simulink model "Computer"  (R2023a)
settings: Solver=VariableStepDiscrete  StartTime=0.0  StopTime=inf  RelTol=1e-3  EnableMultiTasking=on
values from neighbouring files (symbols this model uses):
  RomCode = Preprocessor(RomCode, c)    [ROM.m]
undefined symbols (not defined in the file or in its folder): c, in, RomCodeBreakpoints, RomData, RomDataBreakpoints, UartDataRx, UartDataRx_Active
libraries: Miscellaneous x281, simulink_extras x66, Memory_Blocks_Lib x46, simulink x42, Word_Multiplexers_Lib x31, Decoders_Lib x30, Encoders_Lib x10, Counters_Lib x9, Bit_Multiplexers_Lib x8, Arithmetic_Operations_Lib x5, Bit_Demultiplexers_Lib x4, Garbage x1
(part 4 of 6)

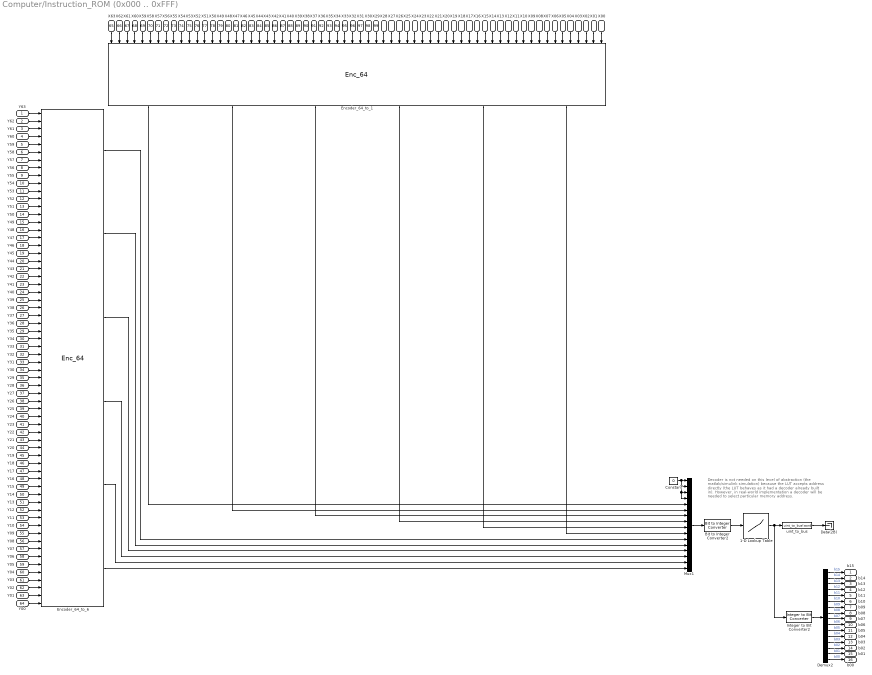
== system Computer/Instruction_ROM (0x000 .. 0xFFF) ==
  note: Decoder is not needed on this level of abstraction (the matlab/simulink simulation) because the LUT accepts address directly (the LUT behaves as it had a decoder already built in). However, in real-world implementation a decoder will be needed to select particular memory address.
  Y63 : Inport
  Y62 : Inport  Port=2
  Y61 : Inport  Port=3
  Y60 : Inport  Port=4
  Y59 : Inport  Port=5
  Y58 : Inport  Port=6
  Y57 : Inport  Port=7
  Y56 : Inport  Port=8
  Y55 : Inport  Port=9
  Y54 : Inport  Port=10
  Y53 : Inport  Port=11
  Y52 : Inport  Port=12
  Y51 : Inport  Port=13
  Y50 : Inport  Port=14
  Y49 : Inport  Port=15
  Y48 : Inport  Port=16
  Y47 : Inport  Port=17
  Y46 : Inport  Port=18
  Y45 : Inport  Port=19
  Y44 : Inport  Port=20
  Y43 : Inport  Port=21
  Y42 : Inport  Port=22
  Y41 : Inport  Port=23
  Y40 : Inport  Port=24
  Y39 : Inport  Port=25
  Y38 : Inport  Port=26
  Y37 : Inport  Port=27
  Y36 : Inport  Port=28
  Y35 : Inport  Port=29
  Y34 : Inport  Port=30
  Y33 : Inport  Port=31
  Y32 : Inport  Port=32
  Y31 : Inport  Port=33
  Y30 : Inport  Port=34
  Y29 : Inport  Port=35
  Y28 : Inport  Port=36
  Y27 : Inport  Port=37
  Y26 : Inport  Port=38
  Y25 : Inport  Port=39
  Y24 : Inport  Port=40
  Y23 : Inport  Port=41
  Y22 : Inport  Port=42
  Y21 : Inport  Port=43
  Y20 : Inport  Port=44
  Y19 : Inport  Port=45
  Y18 : Inport  Port=46
  Y17 : Inport  Port=47
  Y16 : Inport  Port=48
  Y15 : Inport  Port=49
  Y14 : Inport  Port=50
  Y13 : Inport  Port=51
  Y12 : Inport  Port=52
  Y11 : Inport  Port=53
  Y10 : Inport  Port=54
  Y09 : Inport  Port=55
  Y08 : Inport  Port=56
  Y07 : Inport  Port=57
  Y06 : Inport  Port=58
  Y05 : Inport  Port=59
  Y04 : Inport  Port=60
  Y03 : Inport  Port=61
  Y02 : Inport  Port=62
  Y01 : Inport  Port=63
  Y00 : Inport  Port=64
  X63 : Inport  Port=65
  X62 : Inport  Port=66
  X61 : Inport  Port=67
  X60 : Inport  Port=68
  X59 : Inport  Port=69
  X58 : Inport  Port=70
  X57 : Inport  Port=71
  X56 : Inport  Port=72
  X55 : Inport  Port=73
  X54 : Inport  Port=74
  X53 : Inport  Port=75
  X52 : Inport  Port=76
  X51 : Inport  Port=77
  X50 : Inport  Port=78
  X49 : Inport  Port=79
  X48 : Inport  Port=80
  X47 : Inport  Port=81
  X46 : Inport  Port=82
  X45 : Inport  Port=83
  X44 : Inport  Port=84
  X43 : Inport  Port=85
  X42 : Inport  Port=86
  X41 : Inport  Port=87
  X40 : Inport  Port=88
  X39 : Inport  Port=89
  X38 : Inport  Port=90
  X37 : Inport  Port=91
  X36 : Inport  Port=92
  X35 : Inport  Port=93
  X34 : Inport  Port=94
  X33 : Inport  Port=95
  X32 : Inport  Port=96
  X31 : Inport  Port=97
  X30 : Inport  Port=98
  X29 : Inport  Port=99
  X28 : Inport  Port=100
  X27 : Inport  Port=101
  X26 : Inport  Port=102
  X25 : Inport  Port=103
  X24 : Inport  Port=104
  X23 : Inport  Port=105
  X22 : Inport  Port=106
  X21 : Inport  Port=107
  X20 : Inport  Port=108
  X19 : Inport  Port=109
  X18 : Inport  Port=110
  X17 : Inport  Port=111
  X16 : Inport  Port=112
  X15 : Inport  Port=113
  X14 : Inport  Port=114
  X13 : Inport  Port=115
  X12 : Inport  Port=116
  X11 : Inport  Port=117
  X10 : Inport  Port=118
  X09 : Inport  Port=119
  X08 : Inport  Port=120
  X07 : Inport  Port=121
  X06 : Inport  Port=122
  X05 : Inport  Port=123
  X04 : Inport  Port=124
  X03 : Inport  Port=125
  X02 : Inport  Port=126
  X01 : Inport  Port=127
  X00 : Inport  Port=128
  1-D Lookup Table : Lookup_n-D  NumberOfTableDimensions=1  BreakpointsForDimension1=RomCodeBreakpoints  Table=RomCode  InterpMethod=Flat  InternalRulePriority=Speed  RndMeth=Simplest
  Bit to Integer Converter2 : simulink/Logic and Bit Operations/Bit to Integer Converter  nbits=16  bitOrder=MSB first  signedOutputValues=Unsigned  outDtype=uint16  outDtypeSigned=Inherit via internal rule
      settings: LibrarySourceBlock=|
      | commutil2/Bit to Integer
      | Converter
  Constant : Constant  Value=0  OutDataTypeStr=boolean
  Data(2B) : Terminator
  Demux2 : Demux  Outputs=16
  Encoder_64_to_1 : Encoders_Lib/Enc_64  SystemSampleTime=-1  VariantActivationTime=update diagram  Latency=0  AutoFrameSizeCalculation=off
      settings: LibrarySourceBlock=Garbage/Encoder_64_to_6
  Encoder_64_to_6 : Encoders_Lib/Enc_64  SystemSampleTime=-1  VariantActivationTime=update diagram  Latency=0  AutoFrameSizeCalculation=off
      settings: LibrarySourceBlock=Garbage/Encoder_64_to_6
  Integer to Bit Converter2 : simulink/Logic and Bit Operations/Integer to Bit Converter  nbits=16  signedInputValues=Unsigned  bitOrder=MSB first  outDtype=boolean
      settings: LibrarySourceBlock=|
      | commutil2/Integer to Bit
      | Converter
  Mux1 : Mux  Inputs=16
  uint_to_bus : Miscellaneous/uint_to_bus(word)
      settings: LibrarySourceBlock=Miscellaneous/uint_to_bus
  b15 : Outport
  b14 : Outport  Port=2
  b13 : Outport  Port=3
  b12 : Outport  Port=4
  b11 : Outport  Port=5
  b10 : Outport  Port=6
  b09 : Outport  Port=7
  b08 : Outport  Port=8
  b07 : Outport  Port=9
  b06 : Outport  Port=10
  b05 : Outport  Port=11
  b04 : Outport  Port=12
  b03 : Outport  Port=13
  b02 : Outport  Port=14
  b01 : Outport  Port=15
  b00 : Outport  Port=16
  wires:
  1-D Lookup Table/1 -> Integer to Bit Converter2/1, uint_to_bus/1
  Mux1/1 -> Bit to Integer Converter2/1
  uint_to_bus/1 -> Data(2B)/1
  Y04/1 -> Encoder_64_to_6/60
  Y02/1 -> Encoder_64_to_6/62
  Y57/1 -> Encoder_64_to_6/7
  Y07/1 -> Encoder_64_to_6/57
  Y22/1 -> Encoder_64_to_6/42
  Y33/1 -> Encoder_64_to_6/31
  Y54/1 -> Encoder_64_to_6/10
  Y52/1 -> Encoder_64_to_6/12
  Y39/1 -> Encoder_64_to_6/25
  Y19/1 -> Encoder_64_to_6/45
  Y60/1 -> Encoder_64_to_6/4
  Y12/1 -> Encoder_64_to_6/52
  Y44/1 -> Encoder_64_to_6/20
  Y51/1 -> Encoder_64_to_6/13
  Y58/1 -> Encoder_64_to_6/6
  Y16/1 -> Encoder_64_to_6/48
  Y11/1 -> Encoder_64_to_6/53
  Y61/1 -> Encoder_64_to_6/3
  Y32/1 -> Encoder_64_to_6/32
  Y29/1 -> Encoder_64_to_6/35
  Y15/1 -> Encoder_64_to_6/49
  Y21/1 -> Encoder_64_to_6/43
  Y03/1 -> Encoder_64_to_6/61
  Y00/1 -> Encoder_64_to_6/64
  Y23/1 -> Encoder_64_to_6/41
  Y38/1 -> Encoder_64_to_6/26
  Y05/1 -> Encoder_64_to_6/59
  Y01/1 -> Encoder_64_to_6/63
  Y06/1 -> Encoder_64_to_6/58
  Y34/1 -> Encoder_64_to_6/30
  Y08/1 -> Encoder_64_to_6/56
  Y25/1 -> Encoder_64_to_6/39
  Y36/1 -> Encoder_64_to_6/28
  Y59/1 -> Encoder_64_to_6/5
  Y40/1 -> Encoder_64_to_6/24
  Y09/1 -> Encoder_64_to_6/55
  Y42/1 -> Encoder_64_to_6/22
  Y24/1 -> Encoder_64_to_6/40
  Y62/1 -> Encoder_64_to_6/2
  Y30/1 -> Encoder_64_to_6/34
  Y53/1 -> Encoder_64_to_6/11
  Y41/1 -> Encoder_64_to_6/23
  Y35/1 -> Encoder_64_to_6/29
  Y63/1 -> Encoder_64_to_6/1
  Y48/1 -> Encoder_64_to_6/16
  Y55/1 -> Encoder_64_to_6/9
  Y13/1 -> Encoder_64_to_6/51
  Y37/1 -> Encoder_64_to_6/27
  Y45/1 -> Encoder_64_to_6/19
  Y43/1 -> Encoder_64_to_6/21
  Y50/1 -> Encoder_64_to_6/14
  Y27/1 -> Encoder_64_to_6/37
  Y49/1 -> Encoder_64_to_6/15
  Y14/1 -> Encoder_64_to_6/50
  Y18/1 -> Encoder_64_to_6/46
  Y56/1 -> Encoder_64_to_6/8
  Y26/1 -> Encoder_64_to_6/38
  Y31/1 -> Encoder_64_to_6/33
  Y20/1 -> Encoder_64_to_6/44
  Y10/1 -> Encoder_64_to_6/54
  Y17/1 -> Encoder_64_to_6/47
  Y28/1 -> Encoder_64_to_6/36
  Y47/1 -> Encoder_64_to_6/17
  Y46/1 -> Encoder_64_to_6/18
  Constant/1 -> Mux1/2, Mux1/3, Mux1/4, Mux1/1
  X63/1 -> Encoder_64_to_1/1
  X62/1 -> Encoder_64_to_1/2
  X61/1 -> Encoder_64_to_1/3
  X60/1 -> Encoder_64_to_1/4
  X59/1 -> Encoder_64_to_1/5
  X58/1 -> Encoder_64_to_1/6
  X57/1 -> Encoder_64_to_1/7
  X56/1 -> Encoder_64_to_1/8
  X55/1 -> Encoder_64_to_1/9
  X54/1 -> Encoder_64_to_1/10
  X53/1 -> Encoder_64_to_1/11
  X52/1 -> Encoder_64_to_1/12
  X51/1 -> Encoder_64_to_1/13
  X50/1 -> Encoder_64_to_1/14
  X49/1 -> Encoder_64_to_1/15
  X48/1 -> Encoder_64_to_1/16
  X47/1 -> Encoder_64_to_1/17
  X46/1 -> Encoder_64_to_1/18
  X45/1 -> Encoder_64_to_1/19
  X44/1 -> Encoder_64_to_1/20
  X43/1 -> Encoder_64_to_1/21
  X42/1 -> Encoder_64_to_1/22
  X41/1 -> Encoder_64_to_1/23
  X40/1 -> Encoder_64_to_1/24
  X39/1 -> Encoder_64_to_1/25
  X38/1 -> Encoder_64_to_1/26
  X37/1 -> Encoder_64_to_1/27
  X36/1 -> Encoder_64_to_1/28
  X35/1 -> Encoder_64_to_1/29
  X34/1 -> Encoder_64_to_1/30
  X33/1 -> Encoder_64_to_1/31
  X32/1 -> Encoder_64_to_1/32
  X31/1 -> Encoder_64_to_1/33
  X30/1 -> Encoder_64_to_1/34
  X29/1 -> Encoder_64_to_1/35
  X28/1 -> Encoder_64_to_1/36
  X27/1 -> Encoder_64_to_1/37
  X26/1 -> Encoder_64_to_1/38
  X25/1 -> Encoder_64_to_1/39
  X24/1 -> Encoder_64_to_1/40
  X23/1 -> Encoder_64_to_1/41
  X22/1 -> Encoder_64_to_1/42
  X21/1 -> Encoder_64_to_1/43
  X20/1 -> Encoder_64_to_1/44
  X19/1 -> Encoder_64_to_1/45
  X18/1 -> Encoder_64_to_1/46
  X17/1 -> Encoder_64_to_1/47
  X16/1 -> Encoder_64_to_1/48
  X15/1 -> Encoder_64_to_1/49
  X14/1 -> Encoder_64_to_1/50
  X13/1 -> Encoder_64_to_1/51
  X12/1 -> Encoder_64_to_1/52
  X11/1 -> Encoder_64_to_1/53
  X10/1 -> Encoder_64_to_1/54
  X09/1 -> Encoder_64_to_1/55
  X08/1 -> Encoder_64_to_1/56
  X07/1 -> Encoder_64_to_1/57
  X06/1 -> Encoder_64_to_1/58
  X05/1 -> Encoder_64_to_1/59
  X04/1 -> Encoder_64_to_1/60
  X03/1 -> Encoder_64_to_1/61
  X02/1 -> Encoder_64_to_1/62
  X01/1 -> Encoder_64_to_1/63
  X00/1 -> Encoder_64_to_1/64
  Bit to Integer Converter2/1 -> 1-D Lookup Table/1
  Encoder_64_to_6/6 -> Mux1/16
  Encoder_64_to_6/5 -> Mux1/15
  Encoder_64_to_6/4 -> Mux1/14
  Encoder_64_to_6/3 -> Mux1/13
  Encoder_64_to_6/2 -> Mux1/12
  Encoder_64_to_1/1 -> Mux1/5
  Encoder_64_to_1/6 -> Mux1/10
  Encoder_64_to_6/1 -> Mux1/11
  Encoder_64_to_1/5 -> Mux1/9
  Encoder_64_to_1/4 -> Mux1/8
  Encoder_64_to_1/3 -> Mux1/7
  Encoder_64_to_1/2 -> Mux1/6
  Integer to Bit Converter2/1 -> Demux2/1
  Demux2/1 -> b15/1  "b15"
  Demux2/2 -> b14/1  "b14"
  Demux2/3 -> b13/1  "b13"
  Demux2/4 -> b12/1  "b12"
  Demux2/5 -> b11/1  "b11"
  Demux2/6 -> b10/1  "b10"
  Demux2/7 -> b09/1  "b09"
  Demux2/8 -> b08/1  "b08"
  Demux2/9 -> b07/1  "b07"
  Demux2/10 -> b06/1  "b06"
  Demux2/11 -> b05/1  "b05"
  Demux2/12 -> b04/1  "b04"
  Demux2/13 -> b03/1  "b03"
  Demux2/14 -> b02/1  "b02"
  Demux2/15 -> b01/1  "b01"
  Demux2/16 -> b00/1  "b00"

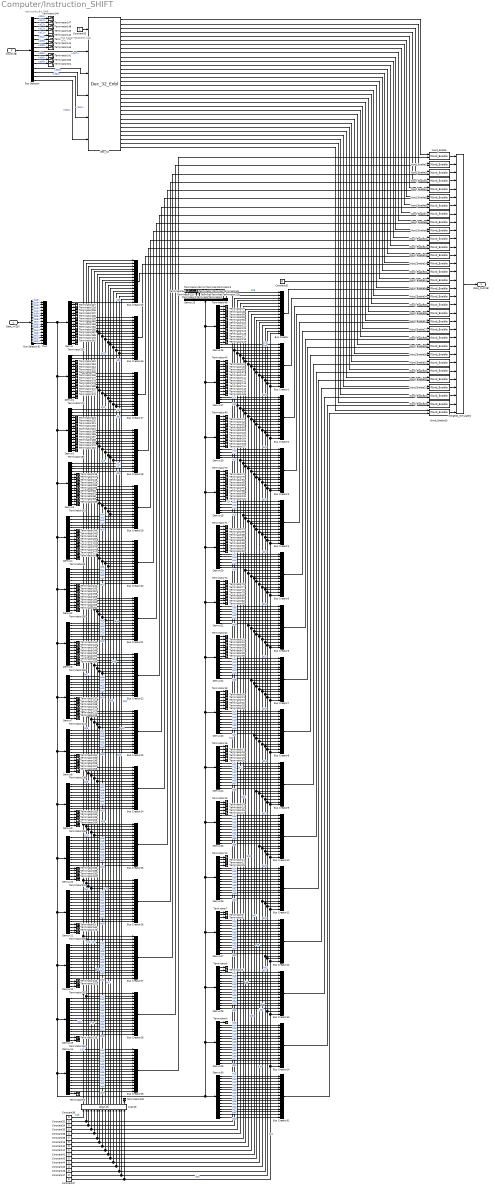
== system Computer/Instruction_SHIFT ==
  note: Instruction_Bit_Shift
  note: This signal
      | represents
      | sign (+/-).
  Data_In(2B) : Inport
  Count(2B) : Inport  Port=2
  Align16 : Miscellaneous/Align16
  Bus Creator{,1..29,31} (31 alike) : BusCreator  Inputs=16
  Bus Selector : BusSelector  OutputSignals=b15,b14,b13,b12,b11,b10,b09,b08,b07,b06,b05,b04,b03,b02,b01,b00
  Bus Selector31 : BusSelector  OutputSignals=b15,b14,b13,b12,b11,b10,b09,b08,b07,b06,b05,b04,b03,b02,b01,b00
  Constant{16,32,34..47} (16 alike) : Constant  Value=0  OutDataTypeStr=boolean
  Constant31 : Constant  Value=0  OutDataTypeStr=Bus: BUS_UINT16_T
  Constant33 : Constant  OutDataTypeStr=boolean
  Dec_32 : Decoders_Lib/Dec_32_Enbl  SystemSampleTime=-1  VariantActivationTime=update diagram  Latency=0  AutoFrameSizeCalculation=off
  Demux{,1..30} (31 alike) : Demux  Outputs=16
  Merge32_Simulated : Miscellaneous/Merge32_Simulated
      settings: LibrarySourceBlock=Memory_Blocks_Lib/Memory_Blocks_Lib/4096x1B_RAM_Simulated
  Mux : Mux  Inputs=16
  Terminator{1..129,140..145,147..153,160..214,216..221,224..272} (252 alike) : Terminator
  Word_Enable{,1..31} (32 alike) : Miscellaneous/Word_Enable  SystemSampleTime=-1  VariantActivationTime=update diagram  Latency=0  AutoFrameSizeCalculation=off
  Data_Out(2B) : Outport
  wires:
  Bus Creator14/1 -> Word_Enable23/2
  Mux/1 -> Demux1/1, Demux2/1, Demux30/1, Demux29/1, Demux24/1, Demux23/1, Demux19/1, Demux18/1, Demux17/1, Demux15/1, Demux16/1, Demux20/1, Demux21/1, Demux22/1, Demux25/1, Demux26/1, Demux27/1, Demux28/1, Demux14/1, Demux13/1, Demux12/1, Demux11/1, Demux10/1, Demux9/1, Demux8/1, Demux7/1, Demux6/1, Demux5/1, Demux4/1, Demux3/1, Demux/1
  Demux29/16 -> Bus Creator14/15  "b01"
  Demux29/15 -> Bus Creator14/14  "b02"
  Demux29/13 -> Bus Creator14/12  "b04"
  Demux29/12 -> Bus Creator14/11  "b05"
  Demux29/11 -> Bus Creator14/10  "b06"
  Demux29/10 -> Bus Creator14/9  "b07"
  Demux29/14 -> Bus Creator14/13  "b03"
  Demux29/9 -> Bus Creator14/8  "b08"
  Demux29/8 -> Bus Creator14/7  "b09"
  Demux29/7 -> Bus Creator14/6  "b10"
  Demux29/6 -> Bus Creator14/5  "b11"
  Demux29/5 -> Bus Creator14/4  "b12"
  Demux29/4 -> Bus Creator14/3  "b13"
  Demux29/3 -> Bus Creator14/2  "b14"
  Demux29/2 -> Bus Creator14/1  "b15"
  Demux29/1 -> Terminator4/1
  Demux28/16 -> Bus Creator13/14  "b02"
  Demux28/15 -> Bus Creator13/13  "b03"
  Demux28/13 -> Bus Creator13/11  "b05"
  Demux28/12 -> Bus Creator13/10  "b06"
  Demux28/11 -> Bus Creator13/9  "b07"
  Demux28/10 -> Bus Creator13/8  "b08"
  Demux28/14 -> Bus Creator13/12  "b04"
  Demux28/9 -> Bus Creator13/7  "b09"
  Demux28/8 -> Bus Creator13/6  "b10"
  Demux28/7 -> Bus Creator13/5  "b11"
  Demux28/6 -> Bus Creator13/4  "b12"
  Demux28/5 -> Bus Creator13/3  "b13"
  Demux28/4 -> Bus Creator13/2  "b14"
  Demux28/3 -> Bus Creator13/1  "b15"
  Demux28/2 -> Terminator6/1
  Demux28/1 -> Terminator5/1
  Bus Creator13/1 -> Word_Enable22/2
  Demux27/16 -> Bus Creator12/13  "b03"
  Demux27/15 -> Bus Creator12/12  "b04"
  Demux27/13 -> Bus Creator12/10  "b06"
  Demux27/12 -> Bus Creator12/9  "b07"
  Demux27/11 -> Bus Creator12/8  "b08"
  Demux27/10 -> Bus Creator12/7  "b09"
  Demux27/14 -> Bus Creator12/11  "b05"
  Demux27/9 -> Bus Creator12/6  "b10"
  Demux27/8 -> Bus Creator12/5  "b11"
  Demux27/7 -> Bus Creator12/4  "b12"
  Demux27/6 -> Bus Creator12/3  "b13"
  Demux27/5 -> Bus Creator12/2  "b14"
  Demux27/4 -> Bus Creator12/1  "b15"
  Demux27/3 -> Terminator9/1
  Demux27/2 -> Terminator8/1
  Demux27/1 -> Terminator7/1
  Bus Creator12/1 -> Word_Enable21/2
  Demux26/16 -> Bus Creator11/12  "b04"
  Demux26/15 -> Bus Creator11/11  "b05"
  Demux26/13 -> Bus Creator11/9  "b07"
  Demux26/12 -> Bus Creator11/8  "b08"
  Demux26/11 -> Bus Creator11/7  "b09"
  Demux26/10 -> Bus Creator11/6  "b10"
  Demux26/14 -> Bus Creator11/10  "b06"
  Demux26/9 -> Bus Creator11/5  "b11"
  Demux26/8 -> Bus Creator11/4  "b12"
  Demux26/7 -> Bus Creator11/3  "b13"
  Demux26/6 -> Bus Creator11/2  "b14"
  Demux26/5 -> Bus Creator11/1  "b15"
  Demux26/3 -> Terminator12/1
  Demux26/2 -> Terminator11/1
  Demux26/1 -> Terminator10/1
  Demux25/16 -> Bus Creator10/11  "b05"
  Demux25/15 -> Bus Creator10/10  "b06"
  Demux25/13 -> Bus Creator10/8  "b08"
  Demux25/12 -> Bus Creator10/7  "b09"
  Demux25/11 -> Bus Creator10/6  "b10"
  Demux25/10 -> Bus Creator10/5  "b11"
  Demux25/14 -> Bus Creator10/9  "b07"
  Demux25/9 -> Bus Creator10/4  "b12"
  Demux25/8 -> Bus Creator10/3  "b13"
  Demux25/7 -> Bus Creator10/2  "b14"
  Demux25/6 -> Bus Creator10/1  "b15"
  Demux25/5 -> Terminator27/1
  Demux25/4 -> Terminator26/1
  Demux25/3 -> Terminator15/1
  Demux25/2 -> Terminator14/1
  Demux25/1 -> Terminator13/1
  Demux24/16 -> Bus Creator9/10  "b06"
  Demux24/15 -> Bus Creator9/9  "b07"
  Demux24/13 -> Bus Creator9/7  "b09"
  Demux24/12 -> Bus Creator9/6  "b10"
  Demux24/11 -> Bus Creator9/5  "b11"
  Demux24/10 -> Bus Creator9/4  "b12"
  Demux24/14 -> Bus Creator9/8  "b08"
  Demux24/9 -> Bus Creator9/3  "b13"
  Demux24/8 -> Bus Creator9/2  "b14"
  Demux24/7 -> Bus Creator9/1  "b15"
  Demux24/6 -> Terminator30/1
  Demux24/5 -> Terminator29/1
  Demux24/4 -> Terminator28/1
  Demux24/3 -> Terminator18/1
  Demux24/2 -> Terminator17/1
  Demux24/1 -> Terminator16/1
  Demux23/16 -> Bus Creator8/9  "b07"
  Demux23/15 -> Bus Creator8/8  "b08"
  Demux23/13 -> Bus Creator8/6  "b10"
  Demux23/12 -> Bus Creator8/5  "b11"
  Demux23/11 -> Bus Creator8/4  "b12"
  Demux23/10 -> Bus Creator8/3  "b13"
  Demux23/14 -> Bus Creator8/7  "b09"
  Demux23/9 -> Bus Creator8/2  "b14"
  Demux23/8 -> Bus Creator8/1  "b15"
  Demux23/7 -> Terminator34/1
  Demux23/6 -> Terminator33/1
  Demux23/5 -> Terminator32/1
  Demux23/4 -> Terminator31/1
  Demux23/3 -> Terminator21/1
  Demux23/2 -> Terminator20/1
  Demux23/1 -> Terminator19/1
  Demux22/16 -> Bus Creator7/8  "b08"
  Demux22/15 -> Bus Creator7/7  "b09"
  Demux22/13 -> Bus Creator7/5  "b11"
  Demux22/12 -> Bus Creator7/4  "b12"
  Demux22/11 -> Bus Creator7/3  "b13"
  Demux22/10 -> Bus Creator7/2  "b14"
  Demux22/14 -> Bus Creator7/6  "b10"
  Demux22/9 -> Bus Creator7/1  "b15"
  Demux22/8 -> Terminator39/1
  Demux22/7 -> Terminator38/1
  Demux22/6 -> Terminator37/1
  Demux22/5 -> Terminator36/1
  Demux22/4 -> Terminator35/1
  Demux22/3 -> Terminator24/1
  Demux22/2 -> Terminator23/1
  Demux22/1 -> Terminator22/1
  Demux26/4 -> Terminator25/1
  Bus Creator11/1 -> Word_Enable20/2
  Bus Creator10/1 -> Word_Enable18/2
  Bus Creator9/1 -> Word_Enable31/2
  Bus Creator8/1 -> Word_Enable30/2
  Bus Creator7/1 -> Word_Enable29/2
  Demux21/16 -> Bus Creator6/7  "b09"
  Demux21/15 -> Bus Creator6/6  "b10"
  Demux21/13 -> Bus Creator6/4  "b12"
  Demux21/12 -> Bus Creator6/3  "b13"
  Demux21/11 -> Bus Creator6/2  "b14"
  Demux21/10 -> Bus Creator6/1  "b15"
  Demux21/14 -> Bus Creator6/5  "b11"
  Demux21/9 -> Terminator83/1
  Demux21/8 -> Terminator82/1
  Demux21/7 -> Terminator81/1
  Demux21/6 -> Terminator80/1
  Demux21/5 -> Terminator79/1
  Demux21/4 -> Terminator78/1
  Demux21/3 -> Terminator77/1
  Demux21/2 -> Terminator76/1
  Demux21/1 -> Terminator70/1
  Demux20/16 -> Bus Creator5/6  "b10"
  Demux20/15 -> Bus Creator5/5  "b11"
  Demux20/13 -> Bus Creator5/3  "b13"
  Demux20/12 -> Bus Creator5/2  "b14"
  Demux20/11 -> Bus Creator5/1  "b15"
  Demux20/10 -> Terminator92/1
  Demux20/14 -> Bus Creator5/4  "b12"
  Demux20/9 -> Terminator91/1
  Demux20/8 -> Terminator90/1
  Demux20/7 -> Terminator89/1
  Demux20/6 -> Terminator88/1
  Demux20/5 -> Terminator87/1
  Demux20/4 -> Terminator86/1
  Demux20/3 -> Terminator85/1
  Demux20/2 -> Terminator72/1
  Demux20/1 -> Terminator71/1
  Demux19/16 -> Bus Creator4/5  "b11"
  Demux19/15 -> Bus Creator4/4  "b12"
  Demux19/13 -> Bus Creator4/2  "b14"
  Demux19/12 -> Bus Creator4/1  "b15"
  Demux19/11 -> Terminator101/1
  Demux19/10 -> Terminator100/1
  Demux19/14 -> Bus Creator4/3  "b13"
  Demux19/9 -> Terminator99/1
  Demux19/8 -> Terminator98/1
  Demux19/7 -> Terminator97/1
  Demux19/6 -> Terminator96/1
  Demux19/5 -> Terminator95/1
  Demux19/4 -> Terminator94/1
  Demux19/3 -> Terminator75/1
  Demux19/2 -> Terminator74/1
  Demux19/1 -> Terminator73/1
  Demux18/16 -> Bus Creator3/4  "b12"
  Demux18/15 -> Bus Creator3/3  "b13"
  Demux18/13 -> Bus Creator3/1  "b15"
  Demux18/12 -> Terminator107/1
  Demux18/11 -> Terminator106/1
  Demux18/10 -> Terminator105/1
  Demux18/14 -> Bus Creator3/2  "b14"
  Demux18/9 -> Terminator104/1
  Demux18/8 -> Terminator103/1
  Demux18/7 -> Terminator102/1
  Demux18/6 -> Terminator93/1
  Demux18/5 -> Terminator84/1
  Demux18/3 -> Terminator42/1
  Demux18/2 -> Terminator41/1
  Demux18/1 -> Terminator40/1
  Demux17/16 -> Bus Creator2/3  "b13"
  Demux17/15 -> Bus Creator2/2  "b14"
  Demux17/13 -> Terminator109/1
  Demux17/12 -> Terminator108/1
  Demux17/11 -> Terminator115/1
  Demux17/10 -> Terminator114/1
  Demux17/14 -> Bus Creator2/1  "b15"
  Demux17/9 -> Terminator113/1
  Demux17/8 -> Terminator112/1
  Demux17/7 -> Terminator111/1
  Demux17/6 -> Terminator110/1
  Demux17/5 -> Terminator57/1
  Demux17/4 -> Terminator56/1
  Demux17/3 -> Terminator45/1
  Demux17/2 -> Terminator44/1
  Demux17/1 -> Terminator43/1
  Demux16/16 -> Bus Creator1/2  "b14"
  Demux16/15 -> Bus Creator1/1  "b15"
  Demux16/13 -> Terminator118/1
  Demux16/12 -> Terminator117/1
  Demux16/11 -> Terminator116/1
  Demux16/10 -> Terminator124/1
  Demux16/14 -> Terminator119/1
  Demux16/9 -> Terminator123/1
  Demux16/8 -> Terminator122/1
  Demux16/7 -> Terminator121/1
  Demux16/6 -> Terminator60/1
  Demux16/5 -> Terminator59/1
  Demux16/4 -> Terminator58/1
  Demux16/3 -> Terminator48/1
  Demux16/2 -> Terminator47/1
  Demux16/1 -> Terminator46/1
  Demux14/16 -> Terminator52/1
  Demux18/4 -> Terminator55/1
  Bus Creator6/1 -> Word_Enable28/2
  Bus Creator5/1 -> Word_Enable27/2
  Bus Creator4/1 -> Word_Enable17/2
  Bus Creator3/1 -> Word_Enable26/2
  Bus Creator2/1 -> Word_Enable25/2
  Bus Creator1/1 -> Word_Enable24/2
  Bus Creator/1 -> Word_Enable16/2
  Bus Creator29/1 -> Word_Enable/2
  Bus Creator28/1 -> Word_Enable2/2
  Bus Creator27/1 -> Word_Enable3/2
  Bus Creator26/1 -> Word_Enable4/2
  Bus Creator25/1 -> Word_Enable1/2
  Bus Creator24/1 -> Word_Enable5/2
  Bus Creator23/1 -> Word_Enable6/2
  Bus Creator22/1 -> Word_Enable7/2
  Bus Creator21/1 -> Word_Enable8/2
  Bus Creator20/1 -> Word_Enable9/2
  Bus Creator19/1 -> Word_Enable10/2
  Bus Creator18/1 -> Word_Enable12/2
  Bus Creator17/1 -> Word_Enable13/2
  Bus Creator16/1 -> Word_Enable14/2
  Bus Creator15/1 -> Word_Enable15/2
  Constant31/1 -> Word_Enable11/2
  Data_In(2B)/1 -> Bus Selector31/1
  Bus Selector31/1 -> Mux/1  "<b15>"
  Bus Selector31/2 -> Mux/2  "<b14>"
  Bus Selector31/4 -> Mux/4  "<b12>"
  Bus Selector31/3 -> Mux/3  "<b13>"
  Bus Selector31/5 -> Mux/5  "<b11>"
  Bus Selector31/6 -> Mux/6  "<b10>"
  Bus Selector31/7 -> Mux/7  "<b09>"
  Bus Selector31/8 -> Mux/8  "<b08>"
  Bus Selector31/9 -> Mux/9  "<b07>"
  Bus Selector31/10 -> Mux/10  "<b06>"
  Bus Selector31/11 -> Mux/11  "<b05>"
  Bus Selector31/12 -> Mux/12  "<b04>"
  Bus Selector31/13 -> Mux/13  "<b03>"
  Bus Selector31/14 -> Mux/14  "<b02>"
  Bus Selector31/15 -> Mux/15  "<b01>"
  Bus Selector31/16 -> Mux/16  "<b00>"
  Demux30/1 -> Bus Creator31/1  "b15"
  Demux30/2 -> Bus Creator31/2  "b14"
  Demux30/4 -> Bus Creator31/4  "b12"
  Demux30/3 -> Bus Creator31/3  "b13"
  Demux30/5 -> Bus Creator31/5  "b11"
  Demux30/6 -> Bus Creator31/6  "b10"
  Demux30/7 -> Bus Creator31/7  "b09"
  Demux30/8 -> Bus Creator31/8  "b08"
  Demux30/9 -> Bus Creator31/9  "b07"
  Demux30/10 -> Bus Creator31/10  "b06"
  Demux30/11 -> Bus Creator31/11  "b05"
  Demux30/12 -> Bus Creator31/12  "b04"
  Demux30/13 -> Bus Creator31/13  "b03"
  Demux30/14 -> Bus Creator31/14  "b02"
  Demux30/15 -> Bus Creator31/15  "b01"
  Demux30/16 -> Bus Creator31/16  "b00"
  Bus Creator31/1 -> Word_Enable19/2
  Dec_32/32 -> Word_Enable19/1
  Dec_32/31 -> Word_Enable23/1
  Dec_32/30 -> Word_Enable22/1
  Dec_32/29 -> Word_Enable21/1
  Dec_32/28 -> Word_Enable20/1
  Dec_32/27 -> Word_Enable18/1
  Dec_32/26 -> Word_Enable31/1
  Dec_32/25 -> Word_Enable30/1
  Dec_32/24 -> Word_Enable29/1
  Dec_32/23 -> Word_Enable28/1
  Dec_32/22 -> Word_Enable27/1
  Dec_32/21 -> Word_Enable17/1
  Dec_32/20 -> Word_Enable26/1
  Dec_32/19 -> Word_Enable25/1
  Dec_32/18 -> Word_Enable24/1
  Dec_32/17 -> Word_Enable16/1
  Dec_32/1 -> Word_Enable/1
  Dec_32/2 -> Word_Enable2/1
  Dec_32/3 -> Word_Enable3/1
  Dec_32/4 -> Word_Enable4/1
  Dec_32/5 -> Word_Enable1/1
  Dec_32/6 -> Word_Enable5/1
  Dec_32/7 -> Word_Enable6/1
  Dec_32/8 -> Word_Enable7/1
  Dec_32/9 -> Word_Enable8/1
  Dec_32/10 -> Word_Enable9/1
  Dec_32/11 -> Word_Enable10/1
  Dec_32/12 -> Word_Enable12/1
  Dec_32/13 -> Word_Enable13/1
  Dec_32/14 -> Word_Enable14/1
  Dec_32/15 -> Word_Enable15/1
  Dec_32/16 -> Word_Enable11/1
  Constant47/1 -> Align16/15, Bus Creator12/15, Bus Creator11/15, Bus Creator10/15, Bus Creator9/15, Bus Creator8/15, Bus Creator7/15, Bus Creator6/15, Bus Creator5/15, Bus Creator4/15, Bus Creator3/15, Bus Creator2/15, Bus Creator1/15, Bus Creator/15, Bus Creator13/15  "b01"
  Constant42/1 -> Align16/10, Bus Creator8/10, Bus Creator7/10, Bus Creator6/10, Bus Creator5/10, Bus Creator4/10, Bus Creator3/10, Bus Creator2/10, Bus Creator1/10, Bus Creator/10  "b06"
  Constant32/1 -> Align16/2, Bus Creator/2  "b14"
  Constant40/1 -> Align16/8, Bus Creator6/8, Bus Creator5/8, Bus Creator4/8, Bus Creator3/8, Bus Creator2/8, Bus Creator1/8, Bus Creator/8  "b08"
  Constant39/1 -> Align16/6, Bus Creator4/6, Bus Creator3/6, Bus Creator2/6, Bus Creator1/6, Bus Creator/6  "b10"
  Constant41/1 -> Align16/9, Bus Creator7/9, Bus Creator6/9, Bus Creator5/9, Bus Creator4/9, Bus Creator3/9, Bus Creator2/9, Bus Creator1/9, Bus Creator/9  "b07"
  Constant34/1 -> Align16/3, Bus Creator1/3, Bus Creator/3  "b13"
  Constant37/1 -> Align16/16, Bus Creator14/16, Bus Creator12/16, Bus Creator11/16, Bus Creator10/16, Bus Creator9/16, Bus Creator8/16, Bus Creator7/16, Bus Creator6/16, Bus Creator5/16, Bus Creator4/16, Bus Creator3/16, Bus Creator2/16, Bus Creator1/16, Bus Creator/16, Bus Creator13/16  "b00"
  Constant38/1 -> Align16/5, Bus Creator3/5, Bus Creator2/5, Bus Creator1/5, Bus Creator/5  "b11"
  Constant35/1 -> Align16/4, Bus Creator2/4, Bus Creator1/4, Bus Creator/4  "b12"
  Constant16/1 -> Align16/7, Bus Creator5/7, Bus Creator4/7, Bus Creator3/7, Bus Creator2/7, Bus Creator1/7, Bus Creator/7  "b09"
  Constant43/1 -> Align16/11, Bus Creator9/11, Bus Creator8/11, Bus Creator7/11, Bus Creator6/11, Bus Creator5/11, Bus Creator4/11, Bus Creator3/11, Bus Creator2/11, Bus Creator1/11, Bus Creator/11  "b05"
  Constant44/1 -> Align16/12, Bus Creator10/12, Bus Creator9/12, Bus Creator8/12, Bus Creator7/12, Bus Creator6/12, Bus Creator5/12, Bus Creator4/12, Bus Creator3/12, Bus Creator2/12, Bus Creator/12, Bus Creator1/12  "b04"
  Constant46/1 -> Align16/14, Bus Creator12/14, Bus Creator11/14, Bus Creator10/14, Bus Creator9/14, Bus Creator8/14, Bus Creator7/14, Bus Creator6/14, Bus Creator5/14, Bus Creator4/14, Bus Creator3/14, Bus Creator2/14, Bus Creator1/14, Bus Creator/14  "b02"
  Constant45/1 -> Align16/13, Bus Creator11/13, Bus Creator10/13, Bus Creator9/13, Bus Creator8/13, Bus Creator7/13, Bus Creator6/13, Bus Creator5/13, Bus Creator4/13, Bus Creator3/13, Bus Creator2/13, Bus Creator1/13, Bus Creator/13  "b03"
  Demux15/7 -> Terminator50/1
  Demux15/1 -> Terminator63/1
  Demux15/6 -> Terminator127/1
  Demux15/5 -> Terminator126/1
  Demux15/4 -> Terminator125/1
  Demux15/10 -> Terminator62/1
  Demux15/11 -> Terminator1/1
  Demux15/12 -> Terminator2/1
  Demux15/8 -> Terminator51/1
  Demux15/2 -> Terminator64/1
  Demux15/9 -> Terminator61/1
  Demux15/14 -> Terminator49/1
  Demux15/3 -> Terminator120/1
  Demux15/13 -> Terminator3/1
  Demux15/15 -> Terminator128/1
  Demux15/16 -> Bus Creator/1  "b15"
  Demux14/7 -> Bus Creator29/8  "b08"
  Demux10/9 -> Bus Creator25/14  "b02"
  Align16/15 -> Bus Creator15/15  "b01"
  Align16/4 -> Bus Creator25/4, Bus Creator24/4, Bus Creator23/4, Bus Creator22/4, Bus Creator21/4, Bus Creator20/4, Bus Creator19/4, Bus Creator18/4, Bus Creator17/4, Bus Creator16/4, Bus Creator15/4, Bus Creator26/4  "b12"
  Demux10/2 -> Bus Creator25/7  "b09"
  Demux8/10 -> Terminator194/1
  Demux6/1 -> Bus Creator21/10  "b06"
  Demux5/15 -> Terminator264/1
  Demux6/6 -> Bus Creator21/15  "b01"
  Demux6/5 -> Bus Creator21/14  "b02"
  Demux13/12 -> Bus Creator28/14  "b02"
  Demux11/7 -> Bus Creator26/11  "b05"
  Demux7/2 -> Bus Creator22/10  "b06"
  Demux7/14 -> Terminator212/1
  Demux8/4 -> Bus Creator23/11  "b05"
  Demux8/2 -> Bus Creator23/9  "b07"
  Demux12/8 -> Bus Creator27/11  "b05"
  Demux7/12 -> Terminator210/1
  Demux7/15 -> Terminator213/1
  Demux6/14 -> Terminator253/1
  Demux7/16 -> Terminator214/1
  Demux8/12 -> Terminator196/1
  Demux13/1 -> Bus Creator28/3  "b13"
  Align16/14 -> Bus Creator16/14, Bus Creator15/14  "b02"
  Demux9/8 -> Bus Creator24/14  "b02"
  Demux9/14 -> Terminator203/1
  Demux9/5 -> Bus Creator24/11  "b05"
  Demux9/11 -> Terminator191/1
  Demux6/11 -> Terminator249/1
  Demux9/13 -> Terminator193/1
  Demux9/15 -> Terminator204/1
  Demux10/6 -> Bus Creator25/11  "b05"
  Demux10/1 -> Bus Creator25/6  "b10"
  Demux10/10 -> Bus Creator25/15  "b01"
  Demux10/8 -> Bus Creator25/13  "b03"
  Demux12/2 -> Bus Creator27/5  "b11"
  Demux11/11 -> Bus Creator26/15  "b01"
  Demux11/6 -> Bus Creator26/10  "b06"
  Demux12/14 -> Terminator240/1
  Demux13/13 -> Bus Creator28/15  "b01"
  Demux12/5 -> Bus Creator27/8  "b08"
  Demux10/11 -> Bus Creator25/16  "b00"
  Demux10/13 -> Terminator189/1
  Demux3/1 -> Bus Creator18/13  "b03"
  Demux11/5 -> Bus Creator26/9  "b07"
  Demux11/10 -> Bus Creator26/14  "b02"
  Demux12/6 -> Bus Creator27/9  "b07"
  Demux2/5 -> Terminator220/1
  Demux2/3 -> Bus Creator17/16  "b00"
  Demux1/10 -> Terminator178/1
  Demux1/15 -> Terminator173/1
  Demux1/14 -> Terminator172/1
  Demux6/7 -> Bus Creator21/16  "b00"
  Demux12/12 -> Bus Creator27/15  "b01"
  Demux6/15 -> Terminator254/1
  Demux1/16 -> Terminator174/1
  Demux2/16 -> Terminator163/1
  Demux7/9 -> Terminator197/1
  Demux2/12 -> Terminator168/1
  Demux2/15 -> Terminator162/1
  Demux10/5 -> Bus Creator25/10  "b06"
  Demux2/9 -> Terminator165/1
  Demux2/11 -> Terminator167/1
  Demux3/2 -> Bus Creator18/14  "b02"
  Demux6/4 -> Bus Creator21/13  "b03"
  Demux6/2 -> Bus Creator21/11  "b05"
  Demux9/7 -> Bus Creator24/13  "b03"
  Demux3/7 -> Terminator218/1
  Demux3/8 -> Terminator229/1
  Demux6/16 -> Terminator255/1
  Demux3/14 -> Terminator69/1
  Demux3/16 -> Terminator161/1
  Demux3/11 -> Terminator66/1
  Demux4/7 -> Terminator245/1
  Demux3/12 -> Terminator67/1
  Demux7/3 -> Bus Creator22/11  "b05"
  Demux3/10 -> Terminator266/1
  Demux3/13 -> Terminator68/1
  Demux4/4 -> Bus Creator19/15  "b01"
  Demux9/2 -> Bus Creator24/8  "b08"
  Demux4/2 -> Bus Creator19/13  "b03"
  Demux14/13 -> Bus Creator29/14  "b02"
  Demux4/3 -> Bus Creator19/14  "b02"
  Demux4/8 -> Terminator246/1
  Demux4/5 -> Bus Creator19/16  "b00"
  Demux5/1 -> Bus Creator20/11  "b05"
  Demux7/5 -> Bus Creator22/13  "b03"
  Demux4/6 -> Terminator244/1
  Align16/3 -> Bus Creator26/3, Bus Creator25/3, Bus Creator24/3, Bus Creator23/3, Bus Creator22/3, Bus Creator21/3, Bus Creator20/3, Bus Creator19/3, Bus Creator18/3, Bus Creator17/3, Bus Creator16/3, Bus Creator15/3, Bus Creator27/3  "b13"
  Demux11/9 -> Bus Creator26/13  "b03"
  Demux5/5 -> Bus Creator20/15  "b01"
  Demux7/1 -> Bus Creator22/9  "b07"
  Demux6/9 -> Terminator247/1
  Demux5/8 -> Terminator243/1
  Demux9/1 -> Bus Creator24/7  "b09"
  Demux5/9 -> Terminator257/1
  Demux7/10 -> Terminator198/1
  Demux10/16 -> Terminator202/1
  Demux5/13 -> Terminator261/1
  Demux8/5 -> Bus Creator23/12  "b04"
  Demux3/9 -> Terminator256/1
  Demux11/8 -> Bus Creator26/12  "b04"
  Align16/5 -> Bus Creator25/5, Bus Creator24/5, Bus Creator23/5, Bus Creator22/5, Bus Creator21/5, Bus Creator20/5, Bus Creator19/5, Bus Creator18/5, Bus Creator17/5, Bus Creator16/5, Bus Creator15/5  "b11"
  Demux1/2 -> Bus Creator16/16  "b00"
  Demux1/4 -> Terminator153/1
  Demux14/6 -> Bus Creator29/7  "b09"
  Demux2/2 -> Bus Creator17/15  "b01"
  Demux8/13 -> Terminator206/1
  Demux4/9 -> Terminator267/1
  Demux12/3 -> Bus Creator27/6  "b10"
  Demux/12 -> Terminator187/1
  Demux1/13 -> Terminator171/1
  Demux2/4 -> Terminator219/1
  Demux12/11 -> Bus Creator27/14  "b02"
  Demux4/11 -> Terminator269/1
  Demux1/12 -> Terminator180/1
  Demux12/7 -> Bus Creator27/10  "b06"
  Demux9/16 -> Terminator205/1
  Demux8/9 -> Bus Creator23/16  "b00"
  Demux12/1 -> Bus Creator27/4  "b12"
  Demux2/6 -> Terminator221/1
  Demux3/3 -> Bus Creator18/15  "b01"
  Demux5/6 -> Bus Creator20/16  "b00"
  Demux7/7 -> Bus Creator22/15  "b01"
  Demux11/15 -> Terminator175/1
  Demux8/15 -> Terminator208/1
  Demux11/12 -> Bus Creator26/16  "b00"
  Demux3/4 -> Bus Creator18/16  "b00"
  Demux/5 -> Terminator237/1
  Demux5/12 -> Terminator260/1
  Demux/6 -> Terminator238/1
  Demux7/4 -> Bus Creator22/12  "b04"
  Demux1/3 -> Terminator152/1
  Demux/8 -> Terminator182/1
  Demux11/14 -> Terminator164/1
  Demux/11 -> Terminator185/1
  Demux8/1 -> Bus Creator23/8  "b08"
  Demux/10 -> Terminator184/1
  Demux4/14 -> Terminator272/1
  Demux3/5 -> Terminator216/1
  Demux/13 -> Terminator188/1
  Demux8/3 -> Bus Creator23/10  "b06"
  Demux8/8 -> Bus Creator23/15  "b01"
  Demux12/4 -> Bus Creator27/7  "b09"
  Demux/15 -> Terminator181/1
  Demux2/1 -> Bus Creator17/14  "b02"
  Demux5/2 -> Bus Creator20/12  "b04"
  Demux1/8 -> Terminator235/1
  Demux11/4 -> Bus Creator26/8  "b08"
  Demux7/11 -> Terminator199/1
  Demux10/15 -> Terminator201/1
  Demux10/12 -> Terminator186/1
  Demux4/13 -> Terminator271/1
  Demux2/13 -> Terminator169/1
  Align16/7 -> Bus Creator23/7, Bus Creator22/7, Bus Creator21/7, Bus Creator20/7, Bus Creator19/7, Bus Creator18/7, Bus Creator17/7, Bus Creator16/7, Bus Creator15/7  "b09"
  Demux13/5 -> Bus Creator28/7  "b09"
  Demux/9 -> Terminator183/1
  Demux13/3 -> Bus Creator28/5  "b11"
  Demux13/15 -> Terminator226/1
  Demux13/6 -> Bus Creator28/8  "b08"
  Demux13/2 -> Bus Creator28/4  "b12"
  Demux13/8 -> Bus Creator28/10  "b06"
  Demux13/14 -> Bus Creator28/16  "b00"
  Demux14/3 -> Bus Creator29/4  "b12"
  Demux14/2 -> Bus Creator29/3  "b13"
  Demux14/5 -> Bus Creator29/6  "b10"
  Demux12/10 -> Bus Creator27/13  "b03"
  Demux12/13 -> Bus Creator27/16  "b00"
  Demux4/12 -> Terminator270/1
  Demux12/15 -> Terminator251/1
  Demux11/3 -> Bus Creator26/7  "b09"
  Demux12/16 -> Terminator262/1
  Align16/9 -> Bus Creator21/9, Bus Creator20/9, Bus Creator19/9, Bus Creator18/9, Bus Creator17/9, Bus Creator16/9, Bus Creator15/9  "b07"
  Demux2/7 -> Terminator230/1
  Demux1/9 -> Terminator177/1
  Align16/2 -> Bus Creator28/2, Bus Creator27/2, Bus Creator26/2, Bus Creator25/2, Bus Creator24/2, Bus Creator23/2, Bus Creator22/2, Bus Creator21/2, Bus Creator20/2, Bus Creator19/2, Bus Creator18/2, Bus Creator17/2, Bus Creator16/2, Bus Creator15/2  "b14"
  Align16/12 -> Bus Creator18/12, Bus Creator17/12, Bus Creator16/12, Bus Creator15/12  "b04"
  Demux9/6 -> Bus Creator24/12  "b04"
  Demux9/10 -> Bus Creator24/16  "b00"
  Demux3/6 -> Terminator217/1
  Demux11/16 -> Terminator200/1
  Demux6/13 -> Terminator252/1
  Demux1/1 -> Bus Creator16/15  "b01"
  Demux1/6 -> Terminator232/1
  Demux4/10 -> Terminator268/1
  Demux8/16 -> Terminator209/1
  Align16/10 -> Bus Creator20/10, Bus Creator19/10, Bus Creator18/10, Bus Creator17/10, Bus Creator16/10, Bus Creator15/10  "b06"
  Align16/11 -> Bus Creator19/11, Bus Creator18/11, Bus Creator17/11, Bus Creator16/11, Bus Creator15/11  "b05"
  Demux6/12 -> Terminator250/1
  Demux6/3 -> Bus Creator21/12  "b04"
  Demux2/8 -> Terminator231/1
  Demux9/12 -> Terminator192/1
  Demux7/13 -> Terminator211/1
  Demux6/10 -> Terminator248/1
  Demux/7 -> Terminator239/1
  Demux14/9 -> Bus Creator29/10  "b06"
  Demux14/4 -> Bus Creator29/5  "b11"
  Demux5/14 -> Terminator263/1
  Demux11/13 -> Terminator53/1
  Demux4/15 -> Terminator54/1
  Demux4/1 -> Bus Creator19/12  "b04"
  Demux1/7 -> Terminator233/1
  Demux10/4 -> Bus Creator25/9  "b07"
  Demux14/8 -> Bus Creator29/9  "b07"
  Demux8/6 -> Bus Creator23/13  "b03"
  Demux14/14 -> Bus Creator29/15  "b01"
  Demux5/10 -> Terminator258/1
  Demux14/12 -> Bus Creator29/13  "b03"
  Demux9/9 -> Bus Creator24/15  "b01"
  Align16/1 -> Bus Creator21/1, Bus Creator20/1, Bus Creator19/1, Bus Creator17/1, Bus Creator15/1, Bus Creator16/1, Bus Creator18/1, Bus Creator22/1, Bus Creator23/1, Bus Creator24/1, Bus Creator25/1, Bus Creator26/1, Bus Creator27/1, Bus Creator28/1, Bus Creator29/1  "b15"
  Demux/16 -> Terminator225/1
  Demux/4 -> Terminator236/1
  Demux5/4 -> Bus Creator20/14  "b02"
  Demux1/5 -> Terminator224/1
  Demux/3 -> Terminator228/1
  Demux5/3 -> Bus Creator20/13  "b03"
  Demux13/10 -> Bus Creator28/12  "b04"
  Demux10/3 -> Bus Creator25/8  "b08"
  Demux14/10 -> Bus Creator29/11  "b05"
  Demux10/14 -> Terminator190/1
  Demux7/8 -> Bus Creator22/16  "b00"
  Demux3/15 -> Terminator160/1
  Demux/14 -> Terminator176/1
  Demux9/4 -> Bus Creator24/10  "b06"
  Demux/2 -> Terminator227/1
  Demux13/11 -> Bus Creator28/13  "b03"
  Demux6/8 -> Terminator241/1
  Demux14/15 -> Bus Creator29/16  "b00"
  Demux2/10 -> Terminator166/1
  Demux/1 -> Bus Creator15/16  "b00"
  Align16/8 -> Bus Creator22/8, Bus Creator21/8, Bus Creator20/8, Bus Creator19/8, Bus Creator18/8, Bus Creator17/8, Bus Creator16/8, Bus Creator15/8  "b08"
  Demux13/4 -> Bus Creator28/6  "b10"
  Demux10/7 -> Bus Creator25/12  "b04"
  Demux14/1 -> Bus Creator29/2  "b14"
  Demux12/9 -> Bus Creator27/12  "b04"
  Demux14/11 -> Bus Creator29/12  "b04"
  Demux8/14 -> Terminator207/1
  Align16/6 -> Bus Creator24/6, Bus Creator23/6, Bus Creator22/6, Bus Creator21/6, Bus Creator20/6, Bus Creator19/6, Bus Creator18/6, Bus Creator17/6, Bus Creator16/6, Bus Creator15/6  "b10"
  Demux8/7 -> Bus Creator23/14  "b02"
  Demux4/16 -> Terminator65/1
  Demux13/16 -> Terminator234/1
  Demux2/14 -> Terminator170/1
  Demux1/11 -> Terminator179/1
  Align16/13 -> Bus Creator17/13, Bus Creator16/13, Bus Creator15/13  "b03"
  Demux8/11 -> Terminator195/1
  Demux7/6 -> Bus Creator22/14  "b02"
  Demux13/7 -> Bus Creator28/9  "b07"
  Demux11/1 -> Bus Creator26/5  "b11"
  Demux5/7 -> Terminator242/1
  Demux11/2 -> Bus Creator26/6  "b10"
  Demux5/16 -> Terminator265/1
  Demux9/3 -> Bus Creator24/9  "b07"
  Demux13/9 -> Bus Creator28/11  "b05"
  Demux5/11 -> Terminator259/1
  Constant36/1 -> Align16/1  "b15"
  Align16/16 -> Terminator129/1
  Bus Selector/13 -> Dec_32/3  "<b03>"
  Bus Selector/9 -> Dec_32/2  "<b07>"
  Bus Selector/4 -> Terminator149/1  "<b12>"
  Bus Selector/3 -> Terminator148/1  "<b13>"
  Count(2B)/1 -> Bus Selector/1
  Bus Selector/12 -> Terminator151/1  "<b04>"
  Bus Selector/8 -> Terminator145/1  "<b08>"
  Bus Selector/11 -> Terminator150/1  "<b05>"
  Bus Selector/10 -> Terminator141/1  "<b06>"
  Bus Selector/6 -> Terminator143/1  "<b10>"
  Bus Selector/16 -> Dec_32/6  "<b00>"
  Bus Selector/2 -> Terminator147/1  "<b14>"
  Bus Selector/14 -> Dec_32/4  "<b02>"
  Bus Selector/15 -> Dec_32/5  "<b01>"
  Bus Selector/7 -> Terminator144/1  "<b09>"
  Bus Selector/1 -> Terminator140/1  "<b15>"
  Bus Selector/5 -> Terminator142/1  "<b11>"
  Constant33/1 -> Dec_32/1
  Word_Enable18/1 -> Merge32_Simulated/27
  Word_Enable23/1 -> Merge32_Simulated/31
  Word_Enable27/1 -> Merge32_Simulated/22
  Word_Enable13/1 -> Merge32_Simulated/13
  Word_Enable4/1 -> Merge32_Simulated/4
  Word_Enable8/1 -> Merge32_Simulated/9
  Word_Enable2/1 -> Merge32_Simulated/2
  Word_Enable15/1 -> Merge32_Simulated/15
  Word_Enable22/1 -> Merge32_Simulated/30
  Word_Enable16/1 -> Merge32_Simulated/17
  Word_Enable14/1 -> Merge32_Simulated/14
  Word_Enable21/1 -> Merge32_Simulated/29
  Word_Enable17/1 -> Merge32_Simulated/21
  Word_Enable/1 -> Merge32_Simulated/1
  Word_Enable29/1 -> Merge32_Simulated/24
  Word_Enable6/1 -> Merge32_Simulated/7
  Word_Enable25/1 -> Merge32_Simulated/19
  Word_Enable3/1 -> Merge32_Simulated/3
  Word_Enable31/1 -> Merge32_Simulated/26
  Word_Enable1/1 -> Merge32_Simulated/5
  Word_Enable28/1 -> Merge32_Simulated/23
  Word_Enable24/1 -> Merge32_Simulated/18
  Word_Enable30/1 -> Merge32_Simulated/25
  Word_Enable19/1 -> Merge32_Simulated/32
  Word_Enable11/1 -> Merge32_Simulated/16
  Word_Enable20/1 -> Merge32_Simulated/28
  Word_Enable12/1 -> Merge32_Simulated/12
  Word_Enable5/1 -> Merge32_Simulated/6
  Word_Enable10/1 -> Merge32_Simulated/11
  Word_Enable7/1 -> Merge32_Simulated/8
  Word_Enable26/1 -> Merge32_Simulated/20
  Word_Enable9/1 -> Merge32_Simulated/10
  Merge32_Simulated/1 -> Data_Out(2B)/1

== system Computer/Instruction_STL ==
  note: Store_Lower_Byte
  Data(2B) : Inport
  Bus Creator : BusCreator  Inputs=16
  Bus Selector : BusSelector  OutputSignals=b07,b06,b05,b04,b03,b02,b01,b00
  Constant{1..3,11..13,15..16} (8 alike) : Constant  Value=0  OutDataTypeStr=boolean
  DataOut(2B) : Outport  OutputWhenDisabled=reset
  wires:
  Data(2B)/1 -> Bus Selector/1
  Bus Creator/1 -> DataOut(2B)/1
  Constant11/1 -> Bus Creator/3  "b13"
  Constant1/1 -> Bus Creator/7  "b09"
  Constant16/1 -> Bus Creator/6  "b10"
  Constant2/1 -> Bus Creator/2  "b14"
  Constant3/1 -> Bus Creator/8  "b08"
  Constant15/1 -> Bus Creator/5  "b11"
  Constant13/1 -> Bus Creator/1  "b15"
  Constant12/1 -> Bus Creator/4  "b12"
  Bus Selector/1 -> Bus Creator/9  "<b07>"
  Bus Selector/2 -> Bus Creator/10  "<b06>"
  Bus Selector/3 -> Bus Creator/11  "<b05>"
  Bus Selector/4 -> Bus Creator/12  "<b04>"
  Bus Selector/5 -> Bus Creator/13  "<b03>"
  Bus Selector/6 -> Bus Creator/14  "<b02>"
  Bus Selector/7 -> Bus Creator/15  "<b01>"
  Bus Selector/8 -> Bus Creator/16  "<b00>"

== system Computer/Instruction_STU ==
  note: Store_Upper_Byte
  Data(2B) : Inport
  Bus Creator : BusCreator  Inputs=16
  Bus Selector1 : BusSelector  OutputSignals=b15,b14,b13,b12,b11,b10,b09,b08
  Constant{1..7,10} (8 alike) : Constant  Value=0  OutDataTypeStr=boolean
  Name{1..7,16} (8 alike) : Miscellaneous/Name
  DataOut(2B) : Outport  OutputWhenDisabled=reset
  wires:
  Data(2B)/1 -> Bus Selector1/1
  Bus Creator/1 -> DataOut(2B)/1
  Name6/1 -> Bus Creator/11  "b05"
  Name16/1 -> Bus Creator/9  "b07"
  Name7/1 -> Bus Creator/16  "b00"
  Name5/1 -> Bus Creator/15  "b01"
  Name4/1 -> Bus Creator/14  "b02"
  Name3/1 -> Bus Creator/13  "b03"
  Name2/1 -> Bus Creator/12  "b04"
  Name1/1 -> Bus Creator/10  "b06"
  Constant10/1 -> Bus Creator/1  "b15"
  Constant1/1 -> Bus Creator/2  "b14"
  Constant3/1 -> Bus Creator/3  "b13"
  Constant2/1 -> Bus Creator/4  "b12"
  Constant5/1 -> Bus Creator/5  "b11"
  Constant4/1 -> Bus Creator/6  "b10"
  Constant7/1 -> Bus Creator/7  "b09"
  Constant6/1 -> Bus Creator/8  "b08"
  Bus Selector1/1 -> Name16/1  "<b15>"
  Bus Selector1/2 -> Name1/1  "<b14>"
  Bus Selector1/3 -> Name6/1  "<b13>"
  Bus Selector1/4 -> Name2/1  "<b12>"
  Bus Selector1/5 -> Name3/1  "<b11>"
  Bus Selector1/6 -> Name4/1  "<b10>"
  Bus Selector1/7 -> Name5/1  "<b09>"
  Bus Selector1/8 -> Name7/1  "<b08>"

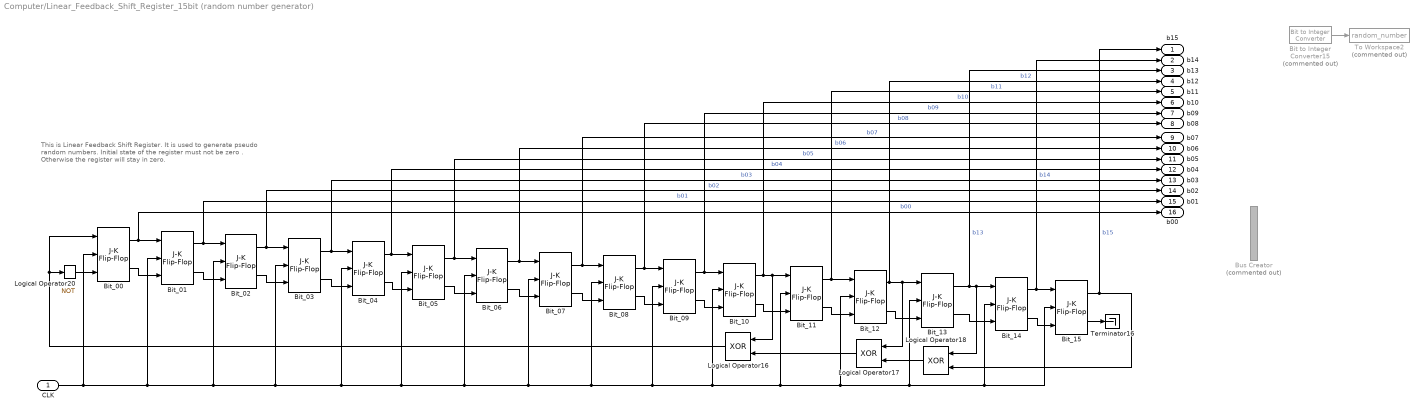
== system Computer/Linear_Feedback_Shift_Register_15bit (random number generator) ==
  note: This is Linear Feedback Shift Register. It is used to generate pseudo random numbers. Initial state of the register must not be zero . Otherwise the register will stay in zero.
  CLK : Inport
  Bit to Integer Converter15 : simulink/Logic and Bit Operations/Bit to Integer Converter  Commented=on  nbits=16  bitOrder=MSB first  signedOutputValues=Unsigned  outDtype=uint16  outDtypeSigned=Inherit via internal rule
      settings: LibrarySourceBlock=|
      | commutil2/Bit to Integer
      | Converter
  Bit_00 : simulink_extras/Flip Flops/J-K Flip-Flop  initial_condition=1
  Bit_01 : simulink_extras/Flip Flops/J-K Flip-Flop  initial_condition=0
  Bit_02 : simulink_extras/Flip Flops/J-K Flip-Flop  initial_condition=0
  Bit_03 : simulink_extras/Flip Flops/J-K Flip-Flop  initial_condition=0
  Bit_04 : simulink_extras/Flip Flops/J-K Flip-Flop  initial_condition=0
  Bit_05 : simulink_extras/Flip Flops/J-K Flip-Flop  initial_condition=0
  Bit_06 : simulink_extras/Flip Flops/J-K Flip-Flop  initial_condition=0
  Bit_07 : simulink_extras/Flip Flops/J-K Flip-Flop  initial_condition=0
  Bit_08 : simulink_extras/Flip Flops/J-K Flip-Flop  initial_condition=0
  Bit_09 : simulink_extras/Flip Flops/J-K Flip-Flop  initial_condition=0
  Bit_{10..15} (6 alike) : simulink_extras/Flip Flops/J-K Flip-Flop  initial_condition=0
  Bus Creator : BusCreator  Commented=on  Inputs=8
  Logical Operator16 : Logic  Operator=XOR  IconShape=distinctive  AllPortsSameDT=off  OutDataTypeStr=boolean
  Logical Operator17 : Logic  Operator=XOR  IconShape=distinctive  AllPortsSameDT=off  OutDataTypeStr=boolean
  Logical Operator18 : Logic  Operator=XOR  IconShape=distinctive  AllPortsSameDT=off  OutDataTypeStr=boolean
  Logical Operator20 : Logic  Operator=NOT  IconShape=distinctive  AllPortsSameDT=off  OutDataTypeStr=boolean
  Terminator16 : Terminator
  To Workspace2 : ToWorkspace  Commented=on  VariableName=random_number  SampleTime=-1
      settings: MaxDataPoints=1  Save2DSignal=2-D array (concatenate along first dimension)
  b15 : Outport
  b14 : Outport  Port=2
  b13 : Outport  Port=3
  b12 : Outport  Port=4
  b11 : Outport  Port=5
  b10 : Outport  Port=6
  b09 : Outport  Port=7
  b08 : Outport  Port=8
  b07 : Outport  Port=9
  b06 : Outport  Port=10
  b05 : Outport  Port=11
  b04 : Outport  Port=12
  b03 : Outport  Port=13
  b02 : Outport  Port=14
  b01 : Outport  Port=15
  b00 : Outport  Port=16
  wires:
  ? -> Bit to Integer Converter15/1
  Bit_11/1 -> b11/1, Bit_12/1  "b11"
  Bit_14/1 -> b14/1, Bit_15/1  "b14"
  Bit_13/1 -> b13/1, Logical Operator18/1, Bit_14/1  "b13"
  Bit_12/1 -> b12/1, Logical Operator17/1, Bit_13/1  "b12"
  Bit_10/1 -> b10/1, Logical Operator16/1, Bit_11/1  "b10"
  Bit_09/1 -> b09/1, Bit_10/1  "b09"
  Bit_08/1 -> b08/1, Bit_09/1  "b08"
  Bit_07/1 -> b07/1, Bit_08/1  "b07"
  Bit_06/1 -> b06/1, Bit_07/1  "b06"
  Bit_05/1 -> b05/1, Bit_06/1  "b05"
  Bit_04/1 -> b04/1, Bit_05/1  "b04"
  Bit_03/1 -> b03/1, Bit_04/1  "b03"
  Bit_02/1 -> b02/1, Bit_03/1  "b02"
  Bit_01/1 -> b01/1, Bit_02/1  "b01"
  Bit_15/2 -> Terminator16/1
  Bit_15/1 -> b15/1, Logical Operator18/2  "b15"
  CLK/1 -> Bit_15/2, Bit_14/2, Bit_13/2, Bit_12/2, Bit_11/2, Bit_10/2, Bit_09/2, Bit_08/2, Bit_07/2, Bit_06/2, Bit_05/2, Bit_04/2, Bit_03/2, Bit_02/2, Bit_01/2, Bit_00/2
  Bit_00/1 -> b00/1, Bit_01/1  "b00"
  Bit_11/2 -> Bit_12/3
  Bit_12/2 -> Bit_13/3
  Bit_13/2 -> Bit_14/3
  Bit_08/2 -> Bit_09/3
  Bit_10/2 -> Bit_11/3
  Bit_09/2 -> Bit_10/3
  Bit_07/2 -> Bit_08/3
  Bit_05/2 -> Bit_06/3
  Bit_01/2 -> Bit_02/3
  Bit_03/2 -> Bit_04/3
  Bit_02/2 -> Bit_03/3
  Logical Operator16/1 -> Bit_00/1, Logical Operator20/1
  Bit_00/2 -> Bit_01/3
  Logical Operator17/1 -> Logical Operator16/2
  Logical Operator18/1 -> Logical Operator17/2
  Bit_04/2 -> Bit_05/3
  Bit_06/2 -> Bit_07/3
  Bit_14/2 -> Bit_15/3
  Logical Operator20/1 -> Bit_00/3
  Bit to Integer Converter15/1 -> To Workspace2/1

== system Computer/Majority_Selector (2_out_of_3) ==
  note: Majority_Selector
  B(1b) : Inport
  A(1b) : Inport  Port=2
  C(1b) : Inport  Port=3
  ...then_the_result_depends_only_on_third_bit : Logic  Commented=on  Operator=NAND  IconShape=distinctive  AllPortsSameDT=off  OutDataTypeStr=boolean
  Alignment{,1..3} (4 alike) : Miscellaneous/Alignment  Commented=on  SystemSampleTime=-1  VariantActivationTime=update diagram  Latency=0  AutoFrameSizeCalculation=off
  Are_both_bits_equal? : Logic  Commented=on  Operator=NXOR  IconShape=distinctive  AllPortsSameDT=off  OutDataTypeStr=boolean
  Constant10 : Constant  Commented=on  Value=0  OutDataTypeStr=boolean
  Constant5 : Constant  Commented=on  Value=0  OutDataTypeStr=boolean
  If_equal_then_the_result_depends_on_any_of_them : Logic  Commented=on  Operator=NAND  IconShape=distinctive  AllPortsSameDT=off  OutDataTypeStr=boolean
  If_not_equal... : Logic  Commented=on  Operator=NOT  IconShape=distinctive  AllPortsSameDT=off  OutDataTypeStr=boolean
  Logical Operator1 : Logic  Commented=on  Operator=NOT  IconShape=distinctive  AllPortsSameDT=off  OutDataTypeStr=boolean
  Logical Operator13 : Logic  Commented=on  Operator=NAND  IconShape=distinctive  AllPortsSameDT=off  OutDataTypeStr=boolean
  Logical Operator2 : Logic  Commented=on  Operator=NOT  IconShape=distinctive  AllPortsSameDT=off  OutDataTypeStr=boolean
  Logical Operator4 : Logic  Commented=on  Operator=NOT  IconShape=distinctive  AllPortsSameDT=off  OutDataTypeStr=boolean
  logic{,1..2,7..8} (5 alike) : Logic  Commented=on  Operator=NAND  IconShape=distinctive  AllPortsSameDT=off  OutDataTypeStr=boolean
  logic10 : Logic  Commented=on  Operator=NAND  Inputs=3  IconShape=distinctive  AllPortsSameDT=off  OutDataTypeStr=boolean
  logic3 : Logic  Operator=NAND  IconShape=distinctive  AllPortsSameDT=off  OutDataTypeStr=boolean
  logic4 : Logic  Operator=NAND  IconShape=distinctive  AllPortsSameDT=off  OutDataTypeStr=boolean
  logic5 : Logic  Operator=NAND  IconShape=distinctive  AllPortsSameDT=off  OutDataTypeStr=boolean
  logic6 : Logic  Operator=NAND  Inputs=3  IconShape=distinctive  AllPortsSameDT=off  OutDataTypeStr=boolean
  logic9 : Logic  Commented=on  Operator=NAND  Inputs=3  IconShape=distinctive  AllPortsSameDT=off  OutDataTypeStr=boolean
  D(1b) : Outport
  wires:
  Logical Operator13/1 -> Alignment3/1
  If_equal_then_the_result_depends_on_any_of_them/1 -> Logical Operator13/2
  Are_both_bits_equal?/1 -> If_not_equal.../1, If_equal_then_the_result_depends_on_any_of_them/1
  If_not_equal.../1 -> ...then_the_result_depends_only_on_third_bit/2
  ...then_the_result_depends_only_on_third_bit/1 -> Logical Operator13/1
  Alignment/1 -> ...then_the_result_depends_only_on_third_bit/1
  Alignment1/1 -> Are_both_bits_equal?/1
  Alignment2/1 -> Are_both_bits_equal?/2, If_equal_then_the_result_depends_on_any_of_them/2
  logic6/1 -> D(1b)/1
  Logical Operator1/1 -> logic/1
  Constant5/1 -> logic1/2, Logical Operator1/1
  Logical Operator2/1 -> logic1/1
  Constant10/1 -> Logical Operator2/1, logic/2
  logic/1 -> logic2/1
  logic1/1 -> logic2/2
  A(1b)/1 -> logic3/1, logic4/1
  B(1b)/1 -> logic5/1, logic3/2
  C(1b)/1 -> logic5/2, logic4/2
  logic4/1 -> logic6/2
  logic3/1 -> logic6/1
  logic5/1 -> logic6/3
  logic9/1 -> logic10/3
  logic10/1 -> ?
  logic7/1 -> logic10/1
  ? -> logic7/1, Logical Operator4/1, logic8/1
  Logical Operator4/1 -> logic9/1
  ? -> logic9/3, logic8/2
  ? -> logic7/2, logic9/2
  logic8/1 -> logic10/2
